simulink subsystem "Plateau_tournant"  (R2022a)
settings: Solver=VariableStepAuto  StartTime=0.0  StopTime=10.0  RelTol=1e-3
undefined symbols (not defined in the file or in its folder): Positions, Slots
libraries: vrlib x3, simulink x2
settings Model: Creator=intel  LastModifiedBy=Aalae

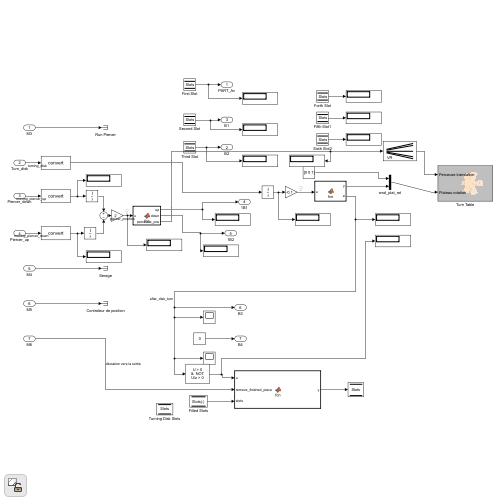
[thumbnail: Simulink's stored preview of the top-level diagram]
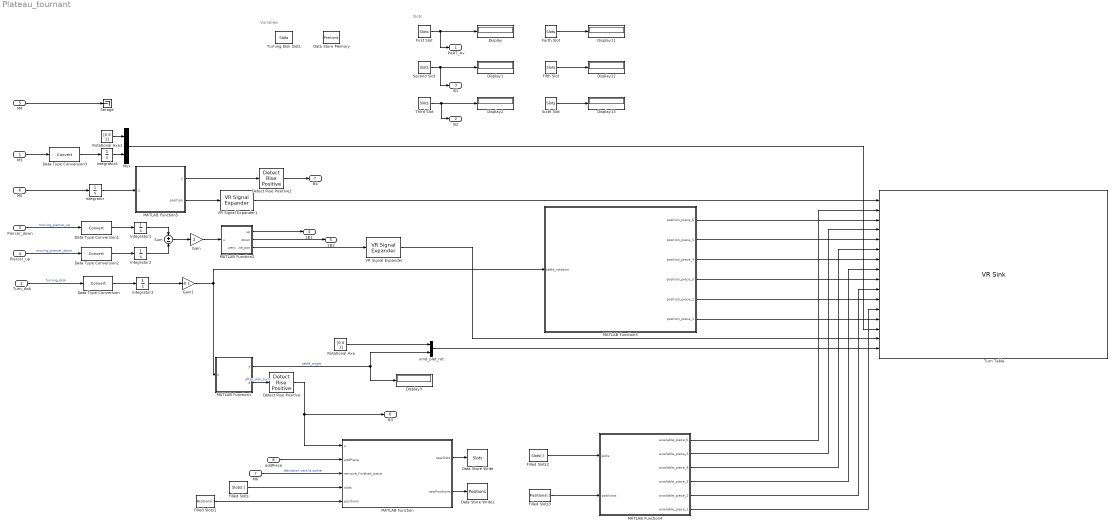
== system Plateau_tournant ==
  note: Variables
  note: Slots
  M3 : Inport
  Turn_disk : Inport  Port=2
  Piercer_down : Inport  Port=3
  Piercer_up : Inport  Port=4
  M4 : Inport  Port=5
  M5 : Inport  Port=6
  M6 : Inport  Port=7
  addPiece : Inport  Port=8
  Data Store Memory : DataStoreMemory  DataStoreName=Positions  WriteAfterWriteMsg=warning  InitialValue=[1,2,3,4,5,6]  ShowAdditionalParam=off
  Data Store Write : DataStoreWrite  DataStoreName=Slots  IndexOptions=Index vector (dialog)  Indices=1  OutputSizes=1
  Data Store Write1 : DataStoreWrite  DataStoreName=Positions  IndexOptions=Index vector (dialog)  Indices=1  OutputSizes=1
  Data Type Conversion{,1..3} (4 alike) : DataTypeConversion  SaturateOnIntegerOverflow=off  RndMeth=Floor
  Detect Rise Positive : simulink/Logic and Bit Operations/Detect Rise Positive  vinit=0  OutDataTypeStr=boolean
  Detect Rise Positive2 : simulink/Logic and Bit Operations/Detect Rise Positive  vinit=0  OutDataTypeStr=boolean
  Display{,1..3,11..13} (7 alike) : Display
  Fifth Slot : DataStoreRead  DataStoreName=Slots  DataStoreElements=Slots  EnableIndexing=on  IndexOptions=Index vector (dialog)  Indices=5  OutputSizes=1
  Filled Slots : DataStoreRead  DataStoreName=Slots  DataStoreElements=Slots(:)  IndexOptions=Index vector (dialog)  Indices=1  OutputSizes=1
  Filled Slots1 : DataStoreRead  DataStoreName=Positions  DataStoreElements=Positions(:)  IndexOptions=Index vector (dialog)  Indices=1  OutputSizes=1
  Filled Slots2 : DataStoreRead  DataStoreName=Slots  DataStoreElements=Slots(:)  IndexOptions=Index vector (dialog)  Indices=1  OutputSizes=1
  Filled Slots3 : DataStoreRead  DataStoreName=Positions  DataStoreElements=Positions(:)  IndexOptions=Index vector (dialog)  Indices=1  OutputSizes=1
  First Slot : DataStoreRead  DataStoreName=Slots  DataStoreElements=Slots  EnableIndexing=on  IndexOptions=Index vector (dialog)  Indices=1  OutputSizes=1
  Forth Slot : DataStoreRead  DataStoreName=Slots  DataStoreElements=Slots  EnableIndexing=on  IndexOptions=Index vector (dialog)  Indices=4  OutputSizes=1
  Gain : Gain  Gain=2
  Gain1 : Gain  Gain=-0.1
  Integrator{,1..4} (5 alike) : Integrator
  MATLAB Function : MATLAB Function  TreatAsAtomicUnit=on
  MATLAB Function1 : MATLAB Function  TreatAsAtomicUnit=on
  MATLAB Function2 : MATLAB Function  TreatAsAtomicUnit=on
  MATLAB Function3 : MATLAB Function  TreatAsAtomicUnit=on
  MATLAB Function4 : MATLAB Function  TreatAsAtomicUnit=on
  MATLAB Function5 : MATLAB Function  TreatAsAtomicUnit=on
  Mux : Mux  Inputs=2
  Rotational Axe : Constant  Value=[0 0 1]
  Rotational Axe1 : Constant  Value=[0 0 1]
  Second Slot : DataStoreRead  DataStoreName=Slots  DataStoreElements=Slots  EnableIndexing=on  IndexOptions=Index vector (dialog)  Indices=2  OutputSizes=1
  Serage : Terminator
  Sixth Slot : DataStoreRead  DataStoreName=Slots  DataStoreElements=Slots  EnableIndexing=on  IndexOptions=Index vector (dialog)  Indices=6  OutputSizes=1
  Sum : Sum  Inputs=+|-
  Third Slot : DataStoreRead  DataStoreName=Slots  DataStoreElements=Slots  EnableIndexing=on  IndexOptions=Index vector (dialog)  Indices=3  OutputSizes=1
  Turn Table : vrlib/VR Sink  InstantiateOnLoad=on  SampleTime=0.1  ViewEnable=on  RemoteChange=off  RemoteView=off  FieldsWritten=Position_Controller.translation.3.1.1.double#Piece6.scale.3.1.1.double#Piece6.translation.3.1.1.double#Piece5.scale.3.1.1.double#Piece5.translation.3.1.1.double#Piece4.scale.3.1.1.double#Piece4.translation.3.1.1.double#Piece3.scale.3.1.1.double#Piece3.translation.3.1.1.double#Piece2.scale.3.1.1.double#Piece2.translation.3.1.1.double#Piece1.scale.3.1.1.double#Piece1.translation.3.1.1.double#Perceuse.rotation.4.1.1.double#Perceuse.translation.3.1.1.double#Plateau.rotation.4.1.1.double  WorldFileName=System models\System.wrl  AutoView=off  VideoDimensions=[]  AllowVariableSize=off
  Turning Disk Slots : DataStoreMemory  DataStoreName=Slots  WriteAfterWriteMsg=warning  InitialValue=[true false false false true false]  ShowAdditionalParam=off  OutDataTypeStr=boolean
  VR Signal Expander : vrlib/VR Signal Expander  outwidth=3  outidx=[3]
  VR Signal Expander1 : vrlib/VR Signal Expander  outwidth=3  outidx=[3]
  xmd_plat_rot : Mux  Inputs=2
  PART_Av : Outport
  B2 : Outport  Port=2
  B1 : Outport  Port=3
  1B1 : Outport  Port=4
  1B2 : Outport  Port=5
  B3 : Outport  Port=6
  B4 : Outport  Port=7
  wires:
  MATLAB Function1/2(a) -> Detect Rise Positive/1  "after_disk_turn"
  Filled Slots/1 -> MATLAB Function/4(slots)
  MATLAB Function/1(newSlots) -> Data Store Write/1
  First Slot/1 -> PART_Av/1, Display/1
  Third Slot/1 -> Display2/1, B2/1
  Second Slot/1 -> B1/1, Display1/1
  Turn_disk/1 -> Data Type Conversion/1  "turning_disk"
  M6/1 -> MATLAB Function/3(remove_finished_piece)  "déviation vers la sortie"
  Piercer_down/1 -> Data Type Conversion1/1  "moving_piercer_up"
  Piercer_up/1 -> Data Type Conversion2/1  "moving_piercer_down"
  M4/1 -> Serage/1
  Rotational Axe/1 -> xmd_plat_rot/1
  Integrator3/1 -> Gain1/1
  Data Type Conversion/1 -> Integrator3/1
  MATLAB Function2/2(down) -> 1B2/1
  MATLAB Function2/1(up) -> 1B1/1
  Integrator1/1 -> Sum/1
  Integrator2/1 -> Sum/2
  Data Type Conversion1/1 -> Integrator1/1
  Data Type Conversion2/1 -> Integrator2/1
  Forth Slot/1 -> Display11/1
  Fifth Slot/1 -> Display12/1
  Sixth Slot/1 -> Display13/1
  Gain1/1 -> MATLAB Function1/1(u), MATLAB Function3/1(table_rotation)
  Detect Rise Positive/1 -> B3/1, MATLAB Function/1(u)
  Sum/1 -> Gain/1
  Gain/1 -> MATLAB Function2/1(u)
  MATLAB Function2/3(perceuse_pos) -> VR Signal Expander/1
  addPiece/1 -> MATLAB Function/2(addPiece)
  MATLAB Function1/1(y) -> Display3/1, xmd_plat_rot/2  "table_angle"
  Filled Slots1/1 -> MATLAB Function/5(positions)
  MATLAB Function/2(newPositions) -> Data Store Write1/1
  Filled Slots3/1 -> MATLAB Function4/2(positions)
  Filled Slots2/1 -> MATLAB Function4/1(slots)
  M5/1 -> Integrator/1
  Integrator/1 -> MATLAB Function5/1(u)
  MATLAB Function5/1(y) -> Detect Rise Positive2/1
  MATLAB Function5/2(position) -> VR Signal Expander1/1
  Detect Rise Positive2/1 -> B4/1
  VR Signal Expander1/1 -> Turn Table/1
  MATLAB Function4/1(available_piece_6) -> Turn Table/2
  MATLAB Function3/1(position_piece_6) -> Turn Table/3
  MATLAB Function4/2(available_piece_5) -> Turn Table/4
  MATLAB Function3/2(position_piece_5) -> Turn Table/5
  MATLAB Function4/3(available_piece_4) -> Turn Table/6
  MATLAB Function3/3(position_piece_4) -> Turn Table/7
  MATLAB Function4/4(available_piece_3) -> Turn Table/8
  MATLAB Function3/4(position_piece_3) -> Turn Table/9
  MATLAB Function4/5(available_piece_2) -> Turn Table/10
  MATLAB Function3/5(position_piece_2) -> Turn Table/11
  MATLAB Function4/6(available_piece_1) -> Turn Table/12
  MATLAB Function3/6(position_piece_1) -> Turn Table/13
  VR Signal Expander/1 -> Turn Table/15
  xmd_plat_rot/1 -> Turn Table/16
  Data Type Conversion3/1 -> Integrator4/1
  M3/1 -> Data Type Conversion3/1
  Integrator4/1 -> Mux/2
  Rotational Axe1/1 -> Mux/1
  Mux/1 -> Turn Table/14

== matlab function Plateau_tournant/MATLAB Function1 ==
  data: u input; y output; a output
function [y, a] = fcn(u)
y = u;
a = false;
deg = -pi/3;

if abs(mod(u,deg) - deg)<=0.1
    a=true;
end

== matlab function Plateau_tournant/MATLAB Function ==
  data: u input; addPiece input; remove_finished_piece input; newSlots output; slots input; newPositions output; positions input
function [newSlots,newPositions] = fcn(u, addPiece, remove_finished_piece, slots,positions)

newSlots = slots;
newPositions = positions;

if u
    newSlots = circshift(slots,1);
    newPositions = circshift(positions,-1);
end

if remove_finished_piece
    newSlots(4) = false;
end

if addPiece
    newSlots(1) = true;
end

== matlab function Plateau_tournant/MATLAB Function2 ==
  data: u input; up output; down output; perceuse_pos output
function [up,down,perceuse_pos] = fcn(u)

up = false;
down = false;

u = 40-u;

perceuse_pos = u;

if u >= 40
    up = true;
end

if u <= 15
    down = true;
end

== matlab function Plateau_tournant/MATLAB Function4 ==
  data: available_piece_6 output; available_piece_5 output; available_piece_4 output; available_piece_3 output; available_piece_2 output; slots input; available_piece_1 output; positions input
function [available_piece_6, available_piece_5,available_piece_4,available_piece_3,available_piece_2,available_piece_1]= fcn(slots,positions)

scale =[1,1,1];

available_piece_1 = slots(positions(1))*scale;
available_piece_2 = slots(positions(2))*scale;
available_piece_3 = slots(positions(3))*scale;
available_piece_4 = slots(positions(4))*scale;
available_piece_5 = slots(positions(5))*scale;
available_piece_6 = slots(positions(6))*scale;

== matlab function Plateau_tournant/MATLAB Function3 ==
  data: position_piece_6 output; position_piece_5 output; position_piece_4 output; position_piece_3 output; position_piece_2 output; position_piece_1 output; table_rotation input size=1
function [position_piece_6, position_piece_5,position_piece_4,position_piece_3,position_piece_2,position_piece_1]= fcn(table_rotation)

r=28.5;

position_piece_1 = [r*cos(table_rotation+pi),r*sin(table_rotation+pi),2];
position_piece_2 = [r*cos(table_rotation+2*pi/3),r*sin(table_rotation+2*pi/3),2];
position_piece_3 = [r*cos(table_rotation+pi/3),r*sin(table_rotation+pi/3),2];
position_piece_4 = [r*cos(table_rotation),r*sin(table_rotation),2];
position_piece_5 = [r*cos(table_rotation-pi/3),r*sin(table_rotation-pi/3),2];
position_piece_6 = [r*cos(table_rotation-2*pi/3),r*sin(table_rotation-2*pi/3),2];

== matlab function Plateau_tournant/MATLAB Function5 ==
  data: u input; y output; position output
function [y,position] = fcn(u)

y = 0;
translation = abs(25.5*sin(0.5*u));
position = 40-translation;

if abs(position-40)<=0.5
    y = 1;
    position = 40;
end
